simulink model "two_mass_model"  (R2021b)
settings: Solver=ode8  StartTime=0.0  StopTime=3.0  FixedStep=Tq  RelTol=1e-3
values from neighbouring files (symbols this model uses):
  C = 0.16    [compare_PRs.m]    (also in compare_steps.m; create_training_set.m; rbfnn_ts.mat; rbfnn_ts_4.mat)
  c0 = c_0*1    [calc_PR.m]    (also in rbfnn_ts.mat = 20.6001366722)
  c1 = c_1 + c_0*2*0.001    [calc_PR.m]    (also in rbfnn_ts.mat = 1.04120027334)
  C12 = C12_nom    [calc_params_sensivity.m]    (also in compare_PRs.m = C12_nom*Ttest(3,i); compare_steps.m = C12_nom*Ttest(3,vector_num); create_training_set.m = C12_nom*Ttest(3,i); create_training_set_v2.m = 0.65)
  dec_factor = 20    [create_training_set.m]    (also in rbfnn_ts.mat = 5)
  J1 = J1_nom    [calc_params_sensivity.m]    (also in compare_PRs.m = J1_nom*Ttest(1,i); compare_steps.m = J1_nom*Ttest(1,vector_num); create_training_set.m = J1_nom*Ttest(1,i); create_training_set_v2.m = 0.015)
  J2 = J2_nom    [calc_params_sensivity.m]    (also in compare_PRs.m = J2_nom*Ttest(2,i); compare_steps.m = J2_nom*Ttest(2,vector_num); create_training_set.m = J2_nom*Ttest(2,i); create_training_set_v2.m = 0.05)
  Kd = Kd_v(i)    [calc_params_sensivity.m]    (also in compare_PRs.m = Kd_nom*Ttest(4,i); compare_steps.m = 0.01; create_training_set.m = Kd_nom*Ttest(4,i); create_training_set_v2.m = 0.01)
  Ksp = 7    [compare_PRs.m]    (also in compare_steps.m; create_training_set.m; create_training_set_v2.m = 43.75; rbfnn_ts.mat)
  noise_level = 0    [compare_PRs.m]    (also in create_training_set.m; neuro_net_testing.m)
  pref_gain = 10*(C*c0/Ksp + r0)    [calc_params_sensivity.m]    (also in compare_PRs.m; compare_steps.m; create_training_set.m; neuro_net_testing.m)
  r0 = X(6,1)    [calc_PR.m]    (also in rbfnn_ts.mat = 9.11040776205)
  r1 = X(5,1)    [calc_PR.m]    (also in rbfnn_ts.mat = 1.38670293092)
  r2 = X(4,1)    [calc_PR.m]    (also in rbfnn_ts.mat = 0.695918527374)
  r3 = X(3,1)    [calc_PR.m]    (also in rbfnn_ts.mat = 0.0372641835349)
  Ra = 3.15    [compare_PRs.m]    (also in compare_steps.m; create_training_set.m; rbfnn_ts.mat; rbfnn_ts_4.mat)
  Ta = 0.05    [compare_PRs.m]    (also in compare_steps.m; create_training_set.m; rbfnn_ts.mat; rbfnn_ts_4.mat)
  Tq = 0.01    [create_training_set.m]    (also in create_training_set_v2.m = 0.5; rbfnn_ts.mat; rbfnn_ts_2.mat = 0.5; rbfnn_ts_4.mat = 0.5)
  Uy = 10    [create_training_set.m]
libraries: simulink x1
settings Model: Creator=Ilya  LastModifiedBy=Ilya
settings SolverCC: AlgebraicLoopSolver=TrustRegion
settings DataIOCC: LimitDataPoints=on  SaveFormat=Array  SignalLoggingSaveFormat=ModelDataLogs  ReturnWorkspaceOutputs=off
settings OptimizationCC: BlockReduction=off  BooleanDataType=off  LifeSpan=inf
settings DebuggingCC: SaveWithParameterizedLinksMsg=none  UnderspecifiedInitializationDetection=Classic  MergeDetectMultiDrivingBlocksExec=none  SignalResolutionControl=TryResolveAllWithWarning  MultiTaskDSMMsg=warning  MultiTaskCondExecSysMsg=none  SFUnexpectedBacktrackingDiag=warning  SFNoUnconditionalDefaultTransitionDiag=warning  SFExecutionAtInitializationDiag=none  SFMachineParentedDataDiag=warning  ArithmeticOperatorsInVariantConditions=warning
settings HardwareCC: ProdBitPerPointer=32  ProdBitPerSizeT=32  ProdBitPerPtrDiffT=32  ProdLargestAtomicFloat=None  ProdIntDivRoundTo=Undefined  ProdEndianess=Unspecified  ProdWordSize=32  ProdHWDeviceType=32-bit Generic  TargetUnknown=on
settings ModelReferenceCC: PropagateSignalLabelsOutOfModel=off
settings SFSimCC: SimUseLocalCustomCode=off  CustomCodeUndefinedFunction=UseInterfaceOnly
settings RTWCC: RTWUseLocalCustomCode=off
settings CodeAppCC: StateflowObjectComments=on
settings GRTTargetCC: TargetLangStandard=C89/C90 (ANSI)
settings ConfigComp: CovMetricSettings=dw  CovSaveCumulativeToWorkspaceVar=on  CovSaveSingleToWorkspaceVar=on  CovExternalEMLEnable=off

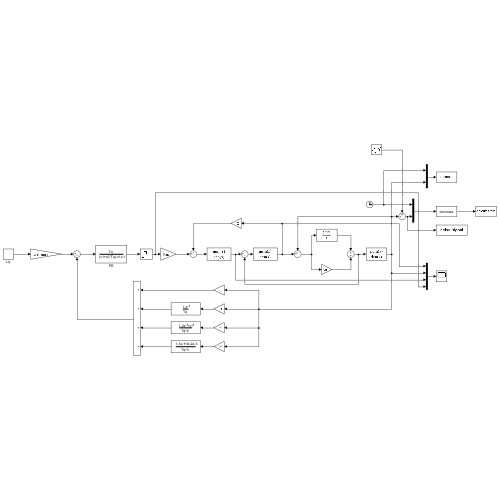
[thumbnail: Simulink's stored preview of the top-level diagram]
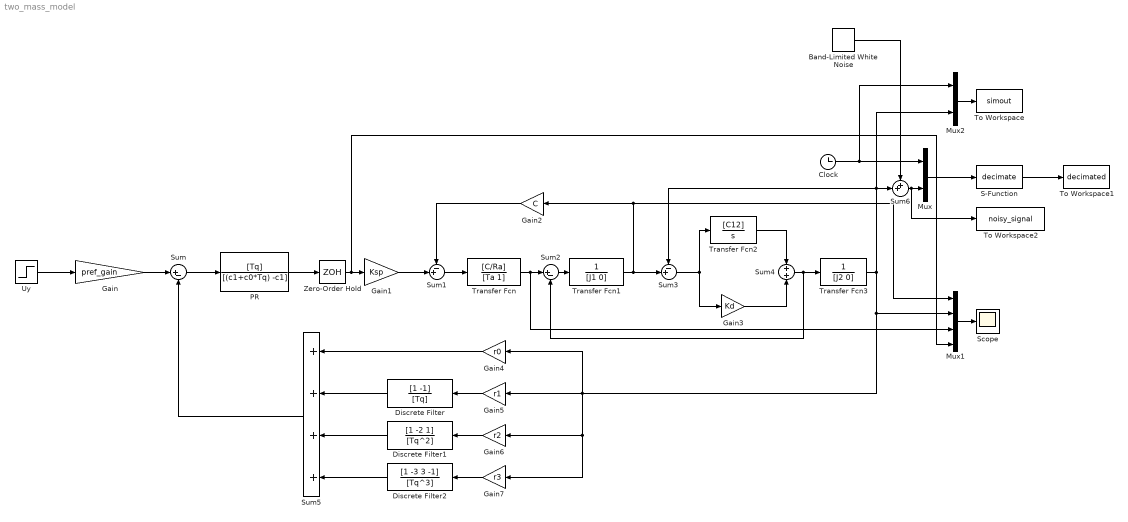
== system two_mass_model ==
  Band-Limited White Noise : simulink/Sources/Band-Limited White Noise  Cov=[noise_level]  Ts=Tq  seed=[23341]
  Clock : Clock
  Discrete Filter : DiscreteFilter  Numerator=[1 -1]  Denominator=[Tq]  SampleTime=Tq
  Discrete Filter1 : DiscreteFilter  Numerator=[1 -2 1]  Denominator=[Tq^2]  SampleTime=Tq
  Discrete Filter2 : DiscreteFilter  Numerator=[1 -3 3 -1]  Denominator=[Tq^3]  SampleTime=Tq
  Gain : Gain  Gain=pref_gain
  Gain1 : Gain  Gain=Ksp
  Gain2 : Gain  Gain=C
  Gain3 : Gain  Gain=Kd
  Gain4 : Gain  Gain=r0  SampleTime=Tq
  Gain5 : Gain  Gain=r1  SampleTime=Tq
  Gain6 : Gain  Gain=r2  SampleTime=Tq
  Gain7 : Gain  Gain=r3  SampleTime=Tq
  Mux : Mux  Inputs=2
  Mux1 : Mux
  Mux2 : Mux  Inputs=2
  PR : DiscreteFilter  Numerator=[Tq]  Denominator=[(c1+c0*Tq) -c1]  SampleTime=Tq
  S-Function : S-Function  FunctionName=decimate  Parameters=Tq,dec_factor,Uy  SFunctionDeploymentMode=off  EnableBusSupport=off
  Scope : Scope
  Sum : Sum  Inputs=|+-
  Sum1 : Sum  Inputs=-+|
  Sum2 : Sum  Inputs=|+-
  Sum3 : Sum  Inputs=-+|
  Sum4 : Sum
  Sum5 : Sum  Inputs=++++  SampleTime=Tq
  Sum6 : Sum  Inputs=++|
  To Workspace : ToWorkspace  VariableName=simout  SampleTime=Tq
  To Workspace1 : ToWorkspace  VariableName=decimated  SampleTime=Tq
      settings: Decimation=dec_factor
  To Workspace2 : ToWorkspace  VariableName=noisy_signal  SampleTime=Tq
  Transfer Fcn : TransferFcn  Numerator=[C/Ra]  Denominator=[Ta 1]
  Transfer Fcn1 : TransferFcn  Denominator=[J1 0]
  Transfer Fcn2 : TransferFcn  Numerator=[C12]  Denominator=[1 0]
  Transfer Fcn3 : TransferFcn  Denominator=[J2 0]
  Uy : Step  Time=0  After=Uy  SampleTime=0
  Zero-Order Hold : ZeroOrderHold  SampleTime=Tq
  wires:
  Uy/1 -> Gain/1
  Gain/1 -> Sum/1
  Sum/1 -> PR/1
  PR/1 -> Zero-Order Hold/1
  Zero-Order Hold/1 -> Mux1/4, Gain1/1
  Gain1/1 -> Sum1/2
  Sum1/1 -> Transfer Fcn/1
  Transfer Fcn/1 -> Mux1/3, Sum2/1
  Sum2/1 -> Transfer Fcn1/1
  Gain2/1 -> Sum1/1
  Transfer Fcn1/1 -> Sum3/2, Mux1/1, Gain2/1
  Sum3/1 -> Transfer Fcn2/1, Gain3/1
  Gain3/1 -> Sum4/2
  Transfer Fcn2/1 -> Sum4/1
  Transfer Fcn3/1 -> Gain6/1, Gain7/1, Gain5/1, Gain4/1, Mux1/2, Mux2/2, Sum3/1, Sum6/2
  Gain4/1 -> Sum5/1
  Gain5/1 -> Discrete Filter/1
  Gain6/1 -> Discrete Filter1/1
  Gain7/1 -> Discrete Filter2/1
  Discrete Filter2/1 -> Sum5/4
  Discrete Filter1/1 -> Sum5/3
  Discrete Filter/1 -> Sum5/2
  Sum5/1 -> Sum/2
  Clock/1 -> Mux2/1, Mux/1
  Mux/1 -> S-Function/1
  S-Function/1 -> To Workspace1/1
  Sum4/1 -> Sum2/2, Transfer Fcn3/1
  Mux1/1 -> Scope/1
  Sum6/1 -> To Workspace2/1, Mux/2
  Band-Limited White Noise/1 -> Sum6/1
  Mux2/1 -> To Workspace/1
